simulink model "model_controller"  (R2024a)
settings: Solver=FixedStepAuto  StartTime=0.0  StopTime=10.0  RelTol=1e-3
undefined symbols (not defined in the file): A, B, C, K, Q, R, x0
settings Model: Creator=anton  LastModifiedBy=anton

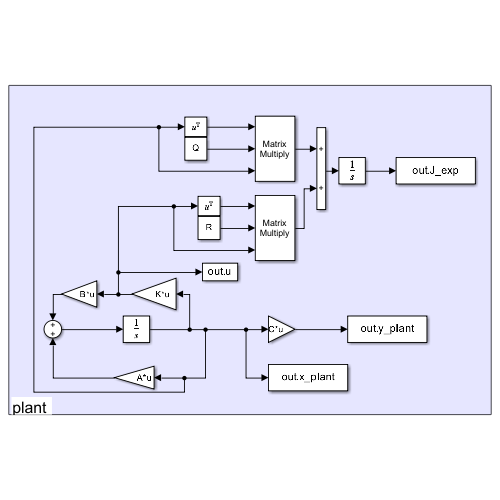
[thumbnail: Simulink's stored preview of the top-level diagram]
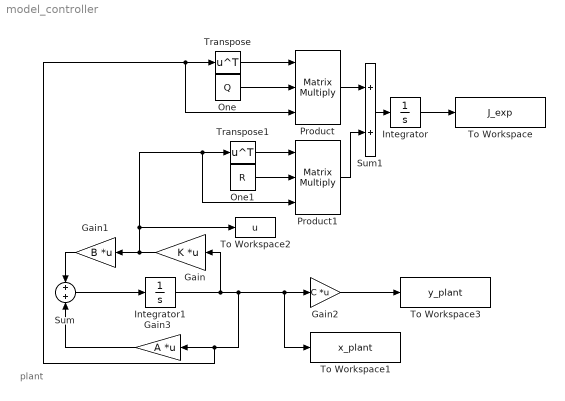
== system model_controller ==
  note: plant
  Gain : Gain  Gain=K  Multiplication=Matrix(K*u)
  Gain1 : Gain  Gain=B  Multiplication=Matrix(K*u)
  Gain2 : Gain  Gain=C  Multiplication=Matrix(K*u)
  Gain3 : Gain  Gain=A  Multiplication=Matrix(K*u)
  Integrator : Integrator
  Integrator1 : Integrator  InitialCondition=x0
  One : Constant  Value=Q  OutDataTypeStr=Inherit: Inherit via back propagation
  One1 : Constant  Value=R  OutDataTypeStr=Inherit: Inherit via back propagation
  Product : Product  Inputs=3  Multiplication=Matrix(*)
  Product1 : Product  Inputs=3  Multiplication=Matrix(*)
  Sum : Sum
  Sum1 : Sum
  To Workspace : ToWorkspace  VariableName=J_exp  SaveFormat=Timeseries  SampleTime=-1
  To Workspace1 : ToWorkspace  VariableName=x_plant  SaveFormat=Timeseries  SampleTime=-1
  To Workspace2 : ToWorkspace  VariableName=u  SaveFormat=Timeseries  SampleTime=-1
  To Workspace3 : ToWorkspace  VariableName=y_plant  SaveFormat=Timeseries  SampleTime=-1
  Transpose : Math  Operator=transpose
  Transpose1 : Math  Operator=transpose
  wires:
  Integrator1/1 -> Gain/1, Gain3/1, Product/3, Transpose/1, To Workspace1/1, Gain2/1
  Gain2/1 -> To Workspace3/1
  Sum/1 -> Integrator1/1
  Gain/1 -> Product1/3, Transpose1/1, To Workspace2/1, Gain1/1
  Gain3/1 -> Sum/2
  Gain1/1 -> Sum/1
  Product/1 -> Sum1/1
  Transpose/1 -> Product/1
  One/1 -> Product/2
  Product1/1 -> Sum1/2
  Transpose1/1 -> Product1/1
  One1/1 -> Product1/2
  Sum1/1 -> Integrator/1
  Integrator/1 -> To Workspace/1
